simulink model "Task22"  (R2025a)
settings: Solver=VariableStepAuto  StartTime=0.0  StopTime=10.0  RelTol=1e-3
settings Model: Creator=LOQ  LastModifiedBy=LOQ

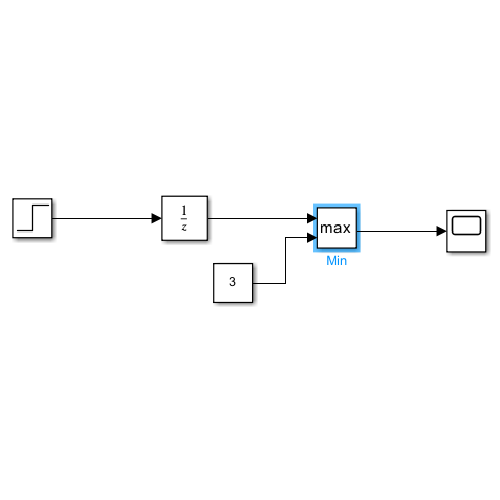
[thumbnail: Simulink's stored preview of the top-level diagram]
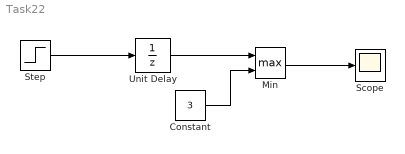
== system Task22 ==
  Constant : Constant  Value=3
  Min : MinMax  Function=max  Inputs=2
  Scope : Scope
      settings: ActiveDisplayYMinimum=-1  ActiveDisplayYMaximum=1
  Step : Step  Time=2  After=10  SampleTime=0
  Unit Delay : UnitDelay  HasFrameUpgradeWarning=on
  wires:
  Step/1 -> Unit Delay/1
  Unit Delay/1 -> Min/1
  Constant/1 -> Min/2
  Min/1 -> Scope/1
